simulink model "GSSA"  (R2015b)
settings: Solver=VariableStepDiscrete  StartTime=0.0  StopTime=45  FixedStep=Ts  RelTol=1e-10  AbsTol=1e-10
values from neighbouring files (symbols this model uses):
  Ts = 0    [Identification.m]    (also in PI_identification_current.m = 0.000125; PI_identification_velocity.m = 0.001; System_Identification.m; The_whole_system_conected.m = 0.001)
undefined symbols (not defined in the file or in its folder): Aser_pf, Bloop_pf, Cloop_pf, DiscIntNeverNeededParam, Dloop_pf
settings Model: Creator=Loki  LastModifiedBy=Loki

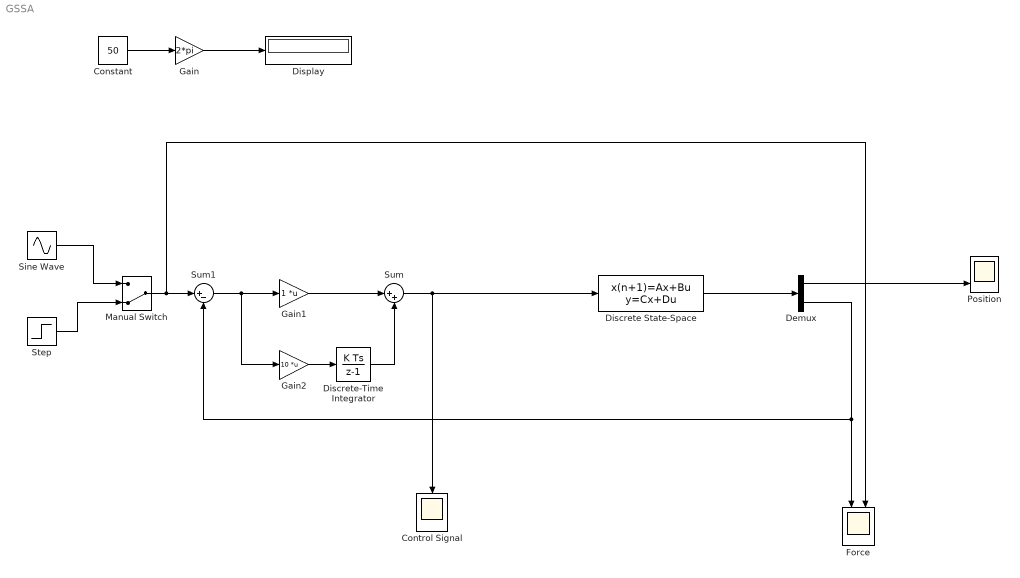
== system GSSA ==
  Constant : Constant  Value=50
  Control Signal : Scope
  Demux : Demux  Outputs=2
  Discrete State-Space : DiscreteStateSpace  A=Aser_pf  B=Bloop_pf  C=Cloop_pf  D=Dloop_pf  SampleTime=Ts
  Discrete-Time Integrator : DiscreteIntegrator  InitialConditionSetting=State (most efficient)  SampleTime=Ts  ICPrevOutput=DiscIntNeverNeededParam  ICPrevScaledInput=DiscIntNeverNeededParam
  Display : Display
  Force : Scope  NumInputPorts=2
  Gain : Gain  Gain=2*pi
  Gain1 : Gain  Multiplication=Matrix(K*u)
  Gain2 : Gain  Gain=10  Multiplication=Matrix(K*u)
  Manual Switch : ManualSwitch  CurrentSetting=0
  "Position " : Scope  NumInputPorts=2
  Sine Wave : Sin  Frequency=314  SampleTime=Ts
  Step : Step  SampleTime=Ts
  Sum : Sum  Inputs=|++
  Sum1 : Sum  Inputs=|+-
  wires:
  Step/1 -> Manual Switch/2
  Sine Wave/1 -> Manual Switch/1
  Manual Switch/1 -> Force/2, Sum1/1
  Demux/1 -> "Position "/2
  Demux/2 -> Sum1/2, Force/1
  Sum1/1 -> Gain2/1, Gain1/1
  Gain/1 -> Display/1
  Constant/1 -> Gain/1
  Sum/1 -> Discrete State-Space/1, Control Signal/1
  Gain1/1 -> Sum/1
  Gain2/1 -> Discrete-Time Integrator/1
  Discrete-Time Integrator/1 -> Sum/2
  Discrete State-Space/1 -> Demux/1
